simulink model "IPILCO_relativeRPY_ST"  (R2014b)
settings: Solver=ode45  StartTime=0.0  StopTime=T  RelTol=1e-3
values from neighbouring files (symbols this model uses):
  dt = 0.01    [settings_ST.m]    (also in settings_ST_puma.m)
  dt_pilco = 0.1    [settings_ST.m]    (also in settings_ST_puma.m)
  indices = 1:1:stateLength    [settings_ST.m]    (also in settings_ST_puma.m)
  initTrial = 0    [learnImp_ST.m]
  jj = J    [learnImp_ST.m]
  Kd_env = [1, 1, 0, 0, 0, 0]    [settings_ST.m]    (also in settings_ST_puma.m)
  Kp_env = [5e3, 5e3, 5e3, 0, 0, 0]    [settings_ST.m]    (also in settings_ST_puma.m = [4e3, 4e3, 0, 0, 0, 0])
  n = robot.n    [settings_ST.m]    (also in settings_ST_puma.m)
  perturbedRobotNF = perturbedRobot.nofriction('all')    [settings_ST.m]    (also in settings_ST_puma.m)
  robot = p560    [settings_ST.m]    (also in settings_ST_puma.m)
  seedMatrix = reshape(seedMatrix,J,[])    [settings_ST.m]    (also in settings_ST_puma.m)
  stateLength = 30    [settings_ST.m]    (also in settings_ST_puma.m)
  xc = [0.45, 0.45, 0.45, 10, 10, 10]'    [settings_ST.m]    (also in settings_ST_puma.m)
  xhole = [0.5, 0.1, 0]    [settings_ST.m]    (also in settings_ST_puma.m = [0.5, 0.2, 0])
undefined symbols (not defined in the file or in its folder): accel, addNoise, cardatol, computeDamping, Hd0, jacob0, jacob_dot, jacobn, plant, policy, q0, tr2rpy, transl, x0trial
libraries: roblocks x10, simulink x1, dspinverses x1
settings Model: Creator=LocalAdmin  LastModifiedBy=LocalAdmin

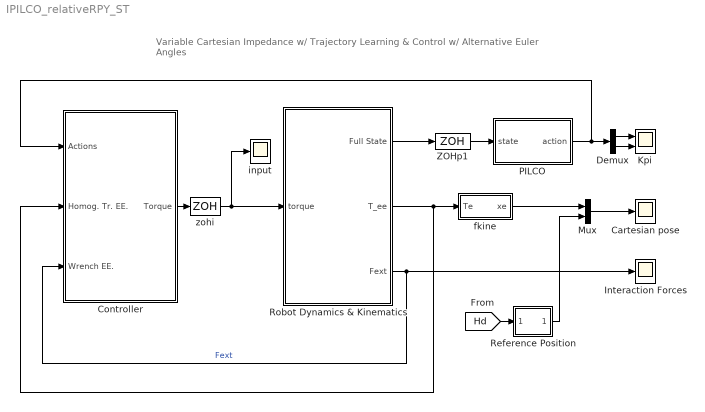
== system IPILCO_relativeRPY_ST ==
  note: Variable Cartesian Impedance w/ Trajectory Learning
      | & Control w/ Alternative Euler Angles
  Cartesian pose : Scope
      settings: TimeRange=0.05  YMin=-0.05  YMax=0.35
  Controller : Subsystem
  Demux : Demux  Outputs=2
  Interaction Forces : Scope
      settings: ShowLegends=on  TimeRange=5  YMin=-35  YMax=10  SaveName=ScopeData2
  Kpi : Scope  NumInputPorts=2
      settings: TimeRange=5  YMin=0~-0.002  YMax=250~0.006  SaveName=ScopeData3
  Mux : Mux  Inputs=2
  PILCO : Subsystem
  Reference Position : Subsystem
  Robot Dynamics & Kinematics : Subsystem
  ZOHp1 : ZeroOrderHold  SampleTime=dt
  fkine : Subsystem
  input : Scope
      settings: ShowLegends=on  TimeRange=0.13  YMin=-1500  YMax=1500  SaveName=ScopeData4
  zohi : ZeroOrderHold  SampleTime=dt
  wires:
  zohi/1 -> Robot Dynamics & Kinematics/1(torque), input/1
  Robot Dynamics & Kinematics/3(Fext) -> Controller/3(Wrench EE.), Interaction Forces/1  "Fext"
  Robot Dynamics & Kinematics/1(Full State) -> ZOHp1/1
  ZOHp1/1 -> PILCO/1(state)
  Controller/1(Torque) -> zohi/1
  Robot Dynamics & Kinematics/2(T_ee) -> Controller/2(Homog. Tr. EE.), fkine/1(Te)
  Reference Position/1(pd) -> Mux/2
  Mux/1 -> Cartesian pose/1
  PILCO/1(action) -> Demux/1, Controller/1(Actions)
  fkine/1(xe) -> Mux/1
  [Hd] -> Reference Position/1(Hd)
  Demux/1 -> Kpi/1
  Demux/2 -> Kpi/2

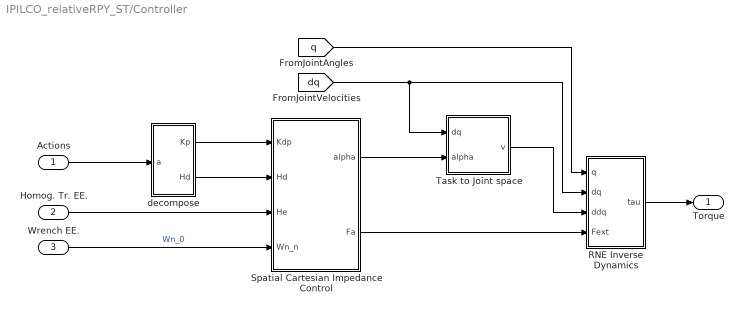
== system IPILCO_relativeRPY_ST/Controller ==
  Actions : Inport
  Homog. Tr. EE. : Inport  Port=2
  Wrench EE. : Inport  Port=3
  RNE Inverse Dynamics : Subsystem
  Spatial Cartesian Impedance Control : Subsystem
  Task to Joint space : Subsystem
  decompose : Subsystem
  Torque : Outport
  wires:
  Spatial Cartesian Impedance Control/1(alpha) -> Task to Joint space/2(alpha)
  Homog. Tr. EE./1 -> Spatial Cartesian Impedance Control/3(He)
  Wrench EE./1 -> Spatial Cartesian Impedance Control/4(Wn_n)  "Wn_0"
  Actions/1 -> decompose/1(a)
  decompose/1(Kp) -> Spatial Cartesian Impedance Control/1(Kdp)
  decompose/2(Hd) -> Spatial Cartesian Impedance Control/2(Hd)
  Task to Joint space/1(v) -> RNE Inverse Dynamics/3(ddq)
  RNE Inverse Dynamics/1(tau) -> Torque/1
  [dq] -> RNE Inverse Dynamics/2(dq), Task to Joint space/1(dq)
  Spatial Cartesian Impedance Control/2(Fa) -> RNE Inverse Dynamics/4(Fext)
  [q] -> RNE Inverse Dynamics/1(q)

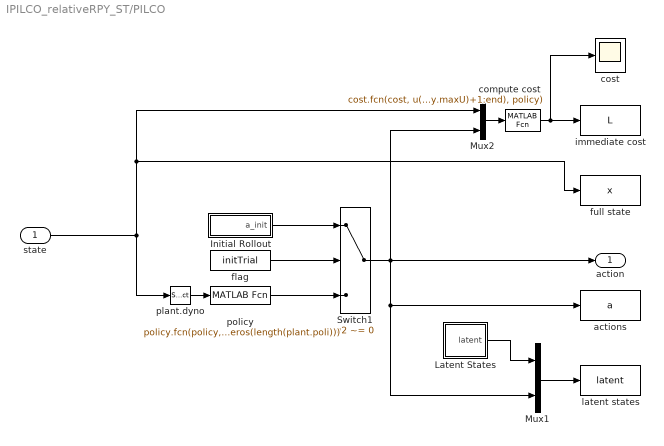
== system IPILCO_relativeRPY_ST/PILCO ==
  state : Inport
  Initial Rollout : Subsystem
  Latent States : Subsystem
  Mux1 : Mux  Inputs=2
  Mux2 : Mux  Inputs=2
  Switch1 : Switch  Criteria=u2 ~= 0
  actions : ToWorkspace  VariableName=a  SampleTime=dt_pilco
  compute cost : MATLABFcn  MATLABFcn=cost.fcn(cost, u(plant.dyno), zeros(length(plant.dyno)), u(end-length(policy.maxU)+1:end), policy)  OutputDimensions=1  Output1D=off
  cost : Scope
      settings: YMin=0  YMax=1.4
  flag : Constant  Value=initTrial  SampleTime=dt_pilco
  full state : ToWorkspace  VariableName=x  SampleTime=dt_pilco
  immediate cost : ToWorkspace  VariableName=L  SampleTime=dt_pilco
  latent states : ToWorkspace  VariableName=latent  SampleTime=dt_pilco
  plant.dyno : Selector  InputPortWidth=length(indices)  Indices=plant.dyno
  policy : MATLABFcn  MATLABFcn=policy.fcn(policy, u(plant.poli), zeros(length(plant.poli)))
  action : Outport
  wires:
  Mux1/1 -> latent states/1
  compute cost/1 -> cost/1, immediate cost/1
  plant.dyno/1 -> policy/1
  Mux2/1 -> compute cost/1
  state/1 -> full state/1, Mux2/1, plant.dyno/1
  Latent States/1(latent) -> Mux1/1
  flag/1 -> Switch1/2
  Initial Rollout/1(a_init) -> Switch1/1
  policy/1 -> Switch1/3
  Switch1/1 -> Mux2/2, Mux1/2, actions/1, action/1

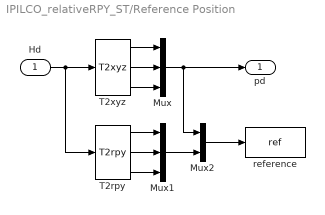
== system IPILCO_relativeRPY_ST/Reference Position ==
  Hd : Inport
  Mux : Mux  Inputs=3
  Mux1 : Mux  Inputs=3
  Mux2 : Mux  Inputs=2
  T2rpy : roblocks/Transform Conversion/T2rpy
  T2xyz : roblocks/Transform Conversion/T2xyz
  reference : ToWorkspace  VariableName=ref  SampleTime=dt_pilco
  pd : Outport
  wires:
  Hd/1 -> T2rpy/1, T2xyz/1
  T2xyz/1 -> Mux/1
  T2xyz/2 -> Mux/2
  T2xyz/3 -> Mux/3
  Mux/1 -> Mux2/1, pd/1
  T2rpy/1 -> Mux1/1
  T2rpy/2 -> Mux1/2
  T2rpy/3 -> Mux1/3
  Mux2/1 -> reference/1
  Mux1/1 -> Mux2/2

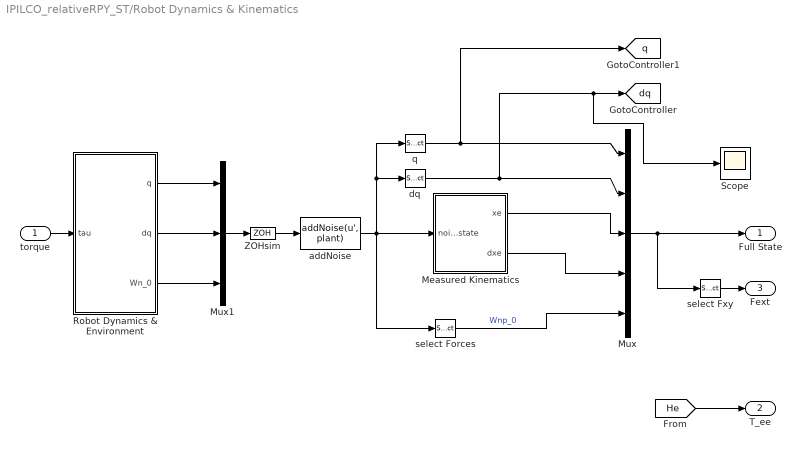
== system IPILCO_relativeRPY_ST/Robot Dynamics & Kinematics ==
  torque : Inport
  Measured Kinematics : Subsystem
  Mux : Mux  Inputs=5
  Mux1 : Mux  Inputs=3
  Robot Dynamics & Environment : Subsystem
  Scope : Scope
      settings: YMin=-80  YMax=60  SaveName=ScopeData7
  ZOHsim : ZeroOrderHold  SampleTime=dt
  addNoise : MATLABFcn  MATLABFcn=addNoise(u', plant)
  dq : Selector  InputPortWidth=2*robot.n+6  Indices=[robot.n+1:2*robot.n]
  q : Selector  InputPortWidth=2*robot.n+6  Indices=[1:robot.n]
  select Forces : Selector  InputPortWidth=2*robot.n+6  Indices=[2*robot.n+1:2*robot.n+6]
  select Fxy : Selector  InputPortWidth=stateLength  Indices=[stateLength-5:1:stateLength]
  Full State : Outport
  T_ee : Outport  Port=2
  Fext : Outport  Port=3
  tag scope: dq=global, q=global
  wires:
  torque/1 -> Robot Dynamics & Environment/1(tau)
  Measured Kinematics/1(xe) -> Mux/3
  Measured Kinematics/2(dxe) -> Mux/4
  select Fxy/1 -> Fext/1
  q/1 -> [q], Mux/1
  dq/1 -> Scope/1, [dq], Mux/2
  Robot Dynamics & Environment/1(q) -> Mux1/1
  Robot Dynamics & Environment/2(dq) -> Mux1/2
  Mux1/1 -> ZOHsim/1
  Robot Dynamics & Environment/3(Wn_0) -> Mux1/3
  Mux/1 -> Full State/1, select Fxy/1
  select Forces/1 -> Mux/5  "Wnp_0"
  [He] -> T_ee/1
  ZOHsim/1 -> addNoise/1
  addNoise/1 -> q/1, dq/1, select Forces/1, Measured Kinematics/1(noisy state)

== system IPILCO_relativeRPY_ST/fkine ==
  Te : Inport
  Mux1 : Mux  Inputs=6
  T2rpy : roblocks/Transform Conversion/T2rpy
  T2xyz : roblocks/Transform Conversion/T2xyz
  xe : Outport
  wires:
  Te/1 -> T2xyz/1, T2rpy/1
  T2xyz/2 -> Mux1/2
  T2rpy/1 -> Mux1/4
  T2xyz/1 -> Mux1/1
  T2rpy/2 -> Mux1/5
  Mux1/1 -> xe/1
  T2xyz/3 -> Mux1/3
  T2rpy/3 -> Mux1/6

== system IPILCO_relativeRPY_ST/Controller/RNE Inverse Dynamics ==
  q : Inport
  dq : Inport  Port=2
  ddq : Inport  Port=3
  Fext : Inport  Port=4
  Mux : Mux
  Recursive Newton-Euler : MATLABFcn  MATLABFcn=rne(robot.nofriction('all'), u(1:n)', u(n+1:2*n)', u(2*n+1:3*n)', robot.gravity', u(3*n+1:end)')  OutputDimensions=n
  tau : Outport
  wires:
  q/1 -> Mux/1
  dq/1 -> Mux/2
  ddq/1 -> Mux/3
  Fext/1 -> Mux/4
  Recursive Newton-Euler/1 -> tau/1
  Mux/1 -> Recursive Newton-Euler/1

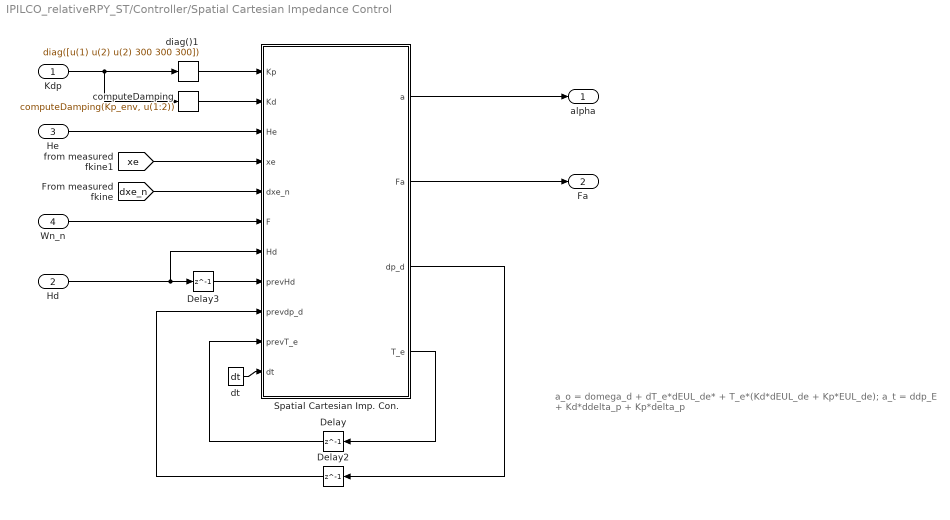
== system IPILCO_relativeRPY_ST/Controller/Spatial Cartesian Impedance Control ==
  note: a_o = domega_d + dT_e*dEUL_de* + T_e*(Kd*dEUL_de + Kp*EUL_de);
      |
      | a_t = ddp_E + Kd*ddelta_p + Kp*delta_p
  Kdp : Inport
  Hd : Inport  Port=2
  He : Inport  Port=3
  Wn_n : Inport  Port=4
  Delay : Delay  DelayLength=1  InitialCondition=cardatol(tr2rpy(Hd0),1,2,3)  SampleTime=dt
  Delay2 : Delay  DelayLength=1  InitialCondition=0  SampleTime=dt
  Delay3 : Delay  DelayLength=1  InitialCondition=Hd0  SampleTime=dt
  Spatial Cartesian Imp. Con. : MATLAB Function  TreatAsAtomicUnit=on
  computeDamping : MATLABFcn  MATLABFcn=computeDamping(Kp_env, u(1:2))  OutputDimensions=[6 6]  Output1D=off
  diag()1 : MATLABFcn  MATLABFcn=diag([u(1) u(2) u(2) 300 300 300])  OutputDimensions=[6 6]  Output1D=off
  dt : Constant  Value=dt  SampleTime=dt
  alpha : Outport
  Fa : Outport  Port=2
  wires:
  Spatial Cartesian Imp. Con./4(T_e) -> Delay/1
  Delay/1 -> Spatial Cartesian Imp. Con./10(prevT_e)
  dt/1 -> Spatial Cartesian Imp. Con./11(dt)
  Hd/1 -> Spatial Cartesian Imp. Con./7(Hd), Delay3/1
  He/1 -> Spatial Cartesian Imp. Con./3(He)
  diag()1/1 -> Spatial Cartesian Imp. Con./1(Kp)
  Spatial Cartesian Imp. Con./3(dp_d) -> Delay2/1
  Delay2/1 -> Spatial Cartesian Imp. Con./9(prevdp_d)
  Delay3/1 -> Spatial Cartesian Imp. Con./8(prevHd)
  [dxe_n] -> Spatial Cartesian Imp. Con./5(dxe_n)
  [xe] -> Spatial Cartesian Imp. Con./4(xe)
  Spatial Cartesian Imp. Con./1(a) -> alpha/1
  computeDamping/1 -> Spatial Cartesian Imp. Con./2(Kd)
  Kdp/1 -> computeDamping/1, diag()1/1
  Wn_n/1 -> Spatial Cartesian Imp. Con./6(F)
  Spatial Cartesian Imp. Con./2(Fa) -> Fa/1

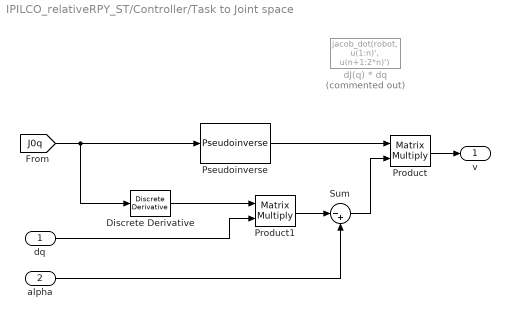
== system IPILCO_relativeRPY_ST/Controller/Task to Joint space ==
  dq : Inport
  alpha : Inport  Port=2
  Discrete Derivative : simulink/Discrete/Discrete Derivative  gainval=1.0  ICPrevScaledInput=0.0  InputProcessing=Inherited  OutMin=[]  OutMax=[]  OutDataType=fixdt(1, 16)  OutScaling=2^-10  DoSatur=off
  Product : Product  Multiplication=Matrix(*)
  Product1 : Product  Multiplication=Matrix(*)
  Pseudoinverse : dspinverses/Pseudoinverse  wanterr=off
  Sum : Sum  Inputs=|-+  SaturateOnIntegerOverflow=on  InputSameDT=on  OutDataTypeStr=Inherit: Same as first input
  dJ(q) * dq : MATLABFcn  Commented=on  MATLABFcn=jacob_dot(robot, u(1:n)', u(n+1:2*n)')  OutputDimensions=[6 1]  Output1D=off
  v : Outport
  wires:
  Discrete Derivative/1 -> Product1/1
  Sum/1 -> Product/2
  Product/1 -> v/1
  Pseudoinverse/1 -> Product/1
  alpha/1 -> Sum/2
  dq/1 -> Product1/2
  [J0q] -> Discrete Derivative/1, Pseudoinverse/1
  Product1/1 -> Sum/1

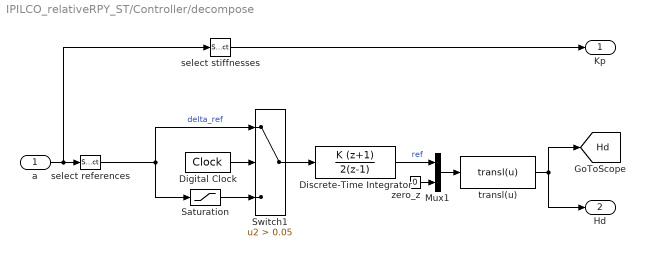
== system IPILCO_relativeRPY_ST/Controller/decompose ==
  a : Inport
  Digital Clock : DigitalClock  SampleTime=dt
  Discrete-Time Integrator : DiscreteIntegrator  IntegratorMethod=Accumulation: Trapezoidal  gainval=1  InitialCondition=x0trial(1:length(policy.refIdx))  InitialConditionSetting=State (most efficient)  SampleTime=-1  LimitOutput=on
  Mux1 : Mux  Inputs=2
  Saturation : Saturate  UpperLimit=0.001  LowerLimit=-0.001
  Switch1 : Switch  Criteria=u2 > Threshold  Threshold=0.05
  select references : Selector  InputPortWidth=length(policy.maxU)  Indices=policy.refIdx
  select stiffnesses : Selector  InputPortWidth=length(policy.maxU)  Indices=policy.impIdx
  transl(u) : MATLABFcn  MATLABFcn=transl(u)  OutputDimensions=[4 4]  Output1D=off
  zero_z : Constant  Value=0  SampleTime=dt
  Kp : Outport
  Hd : Outport  Port=2
  tag scope: Hd=global
  wires:
  select references/1 -> Switch1/1, Saturation/1  "delta_ref"
  select stiffnesses/1 -> Kp/1
  a/1 -> select references/1, select stiffnesses/1
  Discrete-Time Integrator/1 -> Mux1/1  "ref"
  zero_z/1 -> Mux1/2
  transl(u)/1 -> [Hd], Hd/1
  Mux1/1 -> transl(u)/1
  Switch1/1 -> Discrete-Time Integrator/1
  Digital Clock/1 -> Switch1/2
  Saturation/1 -> Switch1/3

== system IPILCO_relativeRPY_ST/PILCO/Initial Rollout ==
  Initial Pos. References : FromWorkspace  VariableName=ainit{jj}  SampleTime=dt  OutputAfterFinalValue=Holding final value
  Mux : Mux  Inputs=2
  Uniform Random Number : UniformRandomNumber  Minimum=policy.minU(policy.impIdx)  Maximum=policy.maxU(policy.impIdx).*2  Seed=seedMatrix(jj,:)  SampleTime=dt_pilco
  XY_des : Selector  InputPortWidth=6  Indices=[1 2]
  a_init : Outport
  wires:
  Initial Pos. References/1 -> XY_des/1
  Uniform Random Number/1 -> Mux/1
  Mux/1 -> a_init/1
  XY_des/1 -> Mux/2

== system IPILCO_relativeRPY_ST/PILCO/Latent States ==
  Mux : Mux  Inputs=5
  latent : Outport
  wires:
  [dq_latent] -> Mux/2
  [q_latent] -> Mux/1
  [wn_0_latent] -> Mux/5
  [dxe_latent] -> Mux/4
  [xe_latent] -> Mux/3
  Mux/1 -> latent/1

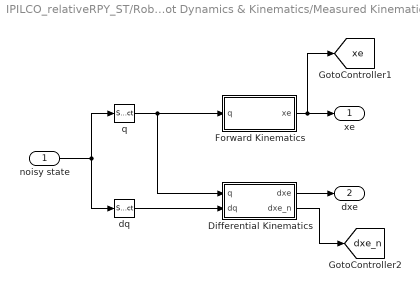
== system IPILCO_relativeRPY_ST/Robot Dynamics & Kinematics/Measured Kinematics ==
  noisy state : Inport
  Differential Kinematics : Subsystem
  Forward Kinematics : Subsystem
  dq : Selector  InputPortWidth=2*robot.n + 6  Indices=[robot.n+1:2*robot.n]
  q : Selector  InputPortWidth=2*robot.n+6  Indices=[1:robot.n]
  xe : Outport
  dxe : Outport  Port=2
  tag scope: dxe_n=global, xe=global
  wires:
  q/1 -> Differential Kinematics/1(q), Forward Kinematics/1(q)
  noisy state/1 -> q/1, dq/1
  dq/1 -> Differential Kinematics/2(dq)
  Differential Kinematics/1(dxe) -> dxe/1
  Forward Kinematics/1(xe) -> [xe], xe/1
  Differential Kinematics/2(dxe_n) -> [dxe_n]

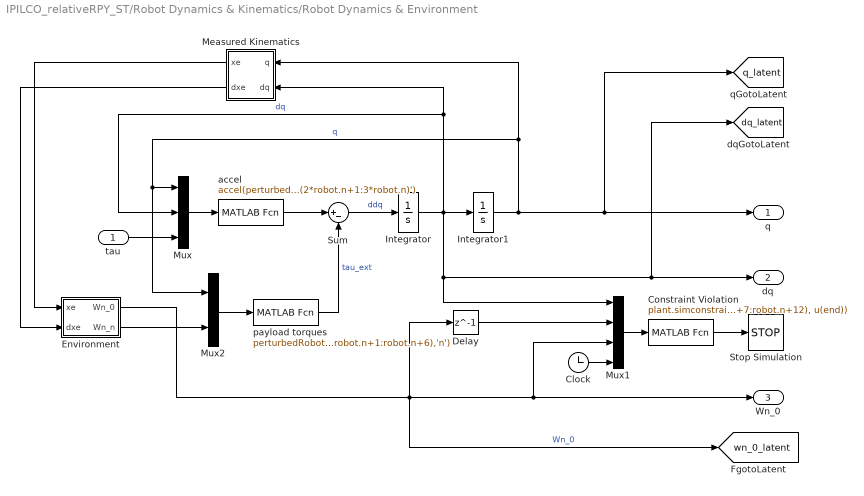
== system IPILCO_relativeRPY_ST/Robot Dynamics & Kinematics/Robot Dynamics & Environment ==
  tau : Inport
  Clock : Clock
  Constraint Violation : MATLABFcn  MATLABFcn=plant.simconstraint(u(1:robot.n), u(robot.n+1:robot.n+6), u(robot.n+7:robot.n+12), u(end))
  Delay : Delay  DelayLength=1  InitialCondition=0  SampleTime=dt
  Environment : Subsystem
  Integrator : Integrator
  Integrator1 : Integrator  InitialCondition=q0
  Measured Kinematics : Subsystem
  Mux : Mux  Inputs=3
  Mux1 : Mux
  Mux2 : Mux  Inputs=2
  Stop Simulation : Stop
  Sum : Sum  Inputs=|+-
  accel : MATLABFcn  MATLABFcn=accel(perturbedRobotNF,u(1:robot.n)',u(robot.n+1:2*robot.n)',u(2*robot.n+1:3*robot.n)')
  payload torques : MATLABFcn  MATLABFcn=perturbedRobotNF.pay(u(1:robot.n)',u(robot.n+1:robot.n+6),'n')
  q : Outport
  dq : Outport  Port=2
  Wn_0 : Outport  Port=3
  tag scope: dq_latent=global, q_latent=global, wn_0_latent=global
  wires:
  accel/1 -> Sum/1
  Mux/1 -> accel/1
  tau/1 -> Mux/3
  payload torques/1 -> Sum/2  "tau_ext"
  Sum/1 -> Integrator/1  "ddq"
  Mux1/1 -> Constraint Violation/1
  Constraint Violation/1 -> Stop Simulation/1
  Measured Kinematics/2(dxe) -> Environment/2(dxe)
  Integrator/1 -> Mux/2, Measured Kinematics/2(dq), Integrator1/1, Mux1/1, [dq_latent], dq/1  "dq"
  Integrator1/1 -> Measured Kinematics/1(q), Mux2/1, Mux/1, [q_latent], q/1  "q"
  Environment/1(Wn_0) -> Delay/1, [wn_0_latent], Mux1/3, Wn_0/1  "Wn_0"
  Mux2/1 -> payload torques/1
  Environment/2(Wn_n) -> Mux2/2
  Measured Kinematics/1(xe) -> Environment/1(xe)
  Delay/1 -> Mux1/2
  Clock/1 -> Mux1/4

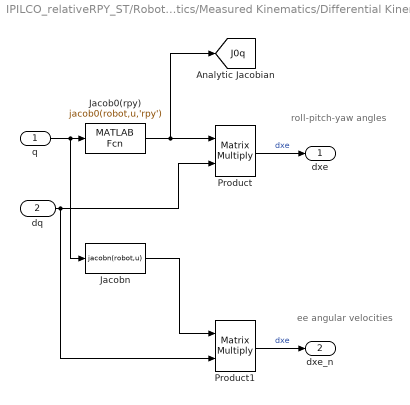
== system IPILCO_relativeRPY_ST/Robot Dynamics & Kinematics/Measured Kinematics/Differential Kinematics ==
  note: roll-pitch-yaw
      | angles
  note: ee angular
      | velocities
  q : Inport
  dq : Inport  Port=2
  Jacob0(rpy) : MATLABFcn  MATLABFcn=jacob0(robot,u,'rpy')  OutputDimensions=[6 n]  Output1D=off
  Jacobn : MATLABFcn  MATLABFcn=jacobn(robot,u)  OutputDimensions=[6 n]  Output1D=off
  Product : Product  Multiplication=Matrix(*)
  Product1 : Product  Multiplication=Matrix(*)
  dxe : Outport
  dxe_n : Outport  Port=2
  tag scope: J0q=global
  wires:
  q/1 -> Jacobn/1, Jacob0(rpy)/1
  Product/1 -> dxe/1  "dxe"
  Jacob0(rpy)/1 -> [J0q], Product/1
  Jacobn/1 -> Product1/1
  Product1/1 -> dxe_n/1  "dxe"
  dq/1 -> Product1/2, Product/2

== system IPILCO_relativeRPY_ST/Robot Dynamics & Kinematics/Measured Kinematics/Forward Kinematics ==
  q : Inport
  Mux : Mux  Inputs=6
  T2rpy : roblocks/Transform Conversion/T2rpy
  T2xyz : roblocks/Transform Conversion/T2xyz
  fkine : roblocks/Kinematics/fkine  robot=robot
  xe : Outport
  tag scope: He=global
  wires:
  T2xyz/3 -> Mux/3
  T2rpy/3 -> Mux/6
  T2rpy/1 -> Mux/4
  T2xyz/2 -> Mux/2
  q/1 -> fkine/1
  fkine/1 -> T2rpy/1, T2xyz/1, [He]
  T2xyz/1 -> Mux/1
  T2rpy/2 -> Mux/5
  Mux/1 -> xe/1

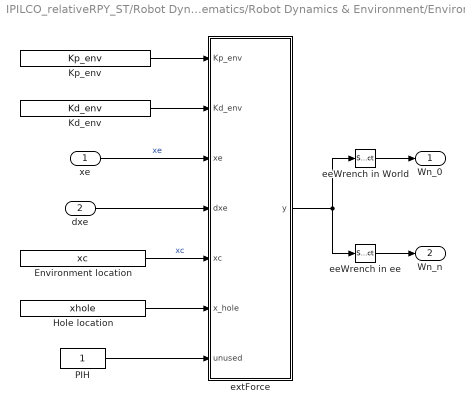
== system IPILCO_relativeRPY_ST/Robot Dynamics & Kinematics/Robot Dynamics & Environment/Environment ==
  xe : Inport
  dxe : Inport  Port=2
  Environment location : Constant  Value=xc  SampleTime=dt
  Hole location : Constant  Value=xhole  SampleTime=dt
  Kd_env : Constant  Value=Kd_env
  Kp_env : Constant  Value=Kp_env
  PIH : Constant  SampleTime=dt
  eeWrench in World : Selector  InputPortWidth=12  Indices=1:1:6
  eeWrench in ee : Selector  InputPortWidth=12  Indices=7:1:12
  extForce : MATLAB Function  TreatAsAtomicUnit=on
  Wn_0 : Outport
  Wn_n : Outport  Port=2
  wires:
  Environment location/1 -> extForce/5(xc)  "xc"
  xe/1 -> extForce/3(xe)  "xe"
  Kp_env/1 -> extForce/1(Kp_env)
  Kd_env/1 -> extForce/2(Kd_env)
  dxe/1 -> extForce/4(dxe)
  extForce/1(y) -> eeWrench in World/1, eeWrench in ee/1
  PIH/1 -> extForce/7(unused)
  eeWrench in World/1 -> Wn_0/1
  eeWrench in ee/1 -> Wn_n/1
  Hole location/1 -> extForce/6(x_hole)

== system IPILCO_relativeRPY_ST/Robot Dynamics & Kinematics/Robot Dynamics & Environment/Measured Kinematics ==
  q : Inport
  dq : Inport  Port=2
  Differential Kinematics : Subsystem
  Forward Kinematics : Subsystem
  xe : Outport
  dxe : Outport  Port=2
  tag scope: dxe_latent=global, xe_latent=global
  wires:
  q/1 -> Differential Kinematics/1(q), Forward Kinematics/1(q)
  dq/1 -> Differential Kinematics/2(dq)
  Differential Kinematics/1(dxe) -> [dxe_latent], dxe/1
  Forward Kinematics/1(xe) -> [xe_latent], xe/1

== system IPILCO_relativeRPY_ST/Robot Dynamics & Kinematics/Robot Dynamics & Environment/Measured Kinematics/Differential Kinematics ==
  q : Inport
  dq : Inport  Port=2
  Jacob0(rpy) : MATLABFcn  MATLABFcn=jacob0(robot,u,'rpy')  OutputDimensions=[6 n]  Output1D=off
  Product : Product  Multiplication=Matrix(*)
  dxe : Outport
  wires:
  q/1 -> Jacob0(rpy)/1
  Product/1 -> dxe/1  "dxe"
  dq/1 -> Product/2
  Jacob0(rpy)/1 -> Product/1

== system IPILCO_relativeRPY_ST/Robot Dynamics & Kinematics/Robot Dynamics & Environment/Measured Kinematics/Forward Kinematics ==
  q : Inport
  Mux : Mux  Inputs=6
  T2rpy : roblocks/Transform Conversion/T2rpy
  T2xyz : roblocks/Transform Conversion/T2xyz
  fkine : roblocks/Kinematics/fkine  robot=robot
  xe : Outport
  wires:
  T2xyz/3 -> Mux/3
  T2rpy/3 -> Mux/6
  T2rpy/1 -> Mux/4
  T2xyz/2 -> Mux/2
  q/1 -> fkine/1
  fkine/1 -> T2rpy/1, T2xyz/1
  T2xyz/1 -> Mux/1
  T2rpy/2 -> Mux/5
  Mux/1 -> xe/1

== matlab function IPILCO_relativeRPY_ST/Controller/Spatial Cartesian Impedance Control/Spatial Cartesian Imp. Con. ==
  data: a output size=[6 1]; Fa output size=[6 1]; dp_d output size=[3 1]; Kp input size=[6 6]; Kd input size=[6 6]; He input size=[4 4]; xe input size=[6 1]; dxe_n input size=[6 1]; F input size=[6 1]; Hd input size=[4 4]; prevHd input size=[4 4]; prevdp_d input size=[3 1]; prevT_e input size=[3 3]; T_e output size=[3 3]; dt input size=1
function [a, Fa, dp_d, T_e] = altEulCartImpControl(Kp, Kd, He, xe, dxe_n, F, Hd, prevHd, prevdp_d, prevT_e, dt)
% Computes modified euler angles EUL_de
%
% Outputs
%               - a             computed impedance actions in Cartesian space
%               - Ta            Transformation between analytical and geometric Jacobian
%               - T_e           transformation of Euler angle deriv. to angular vel. of ee-frame
%               - dT_e          time derivative of transf. matrix.
%
% Inputs:
%               - Kp                diagonal stiffness matrix
%               - Kd                diagonal damping matrix
%               - He                current homog. transf. of ee-frame
%               - Hd                desired homog. transf.
%               - xe                current end-effector pose
%               - dxe_n             current end-effector velocity (ee-frame
%               - prevHd            previous desired homog. transf.
%               - prevdp_d          previous desired translational velocity
%               - prevEUL_de        previous relative euler angles
%               - prevHe            previous homog. transf. of ee-frame
%               - dt                sampling time
%
% Code by Victor van Spaandonk
% May 2016
%

%% Prepare inputs
R_e = tr2rt(He);         % Rotation of ee-frame          (referred to base)
R_d = tr2rt(Hd);          % Rotation of desired frame     (referred to base)

Md = diag([1 1 1 1 1 1]);

%% Translational Actions
p_e = xe(1:3);                  % current ee pos.
p_d = transl(Hd);               % current desired pos.
delta_p = (p_d - p_e);          % positional error

dp_e = dxe_n(1:3);              % current ee transl vel.
prevp_d = transl(prevHd);       % previous desired postion
dp_d = (p_d - prevp_d)./dt;     % current desired velocity
ddelta_p = (dp_d - dp_e);       % velocity error

ddp_d = (dp_d - prevdp_d)./dt;  % current desired acceleration

a_t = ddp_d + inv(Md(1:3,1:3))*(Kd(1:3,1:3)*ddelta_p + Kp(1:3,1:3)*delta_p + F(1:3));

%% Rotational Actions
% EUL_e = my_tr2rpy(R_e,'xyz');           % Euler angles of ee-frame
% Te = cardatol(EUL_e,1,2,3);             % transformation between euler angles derivative and angular velocity of ee-frame
% Ta = [eye(3), zeros(3); zeros(3), Te];  % Transformation relating Geometric and Analytical Jacobian

Re_d = R_e'*R_d;                        % mutual orientation of ee-frame w.r.t. desired frame
EUL_de = my_tr2rpy(Re_d,'xyz')';        % extract EULER rpy-angles (xyz)

T = cardatol(EUL_de,1,2,3);             % Transformation matrix relating Euler angle derivatives to angular velocity      (xyz)
T_e = R_e*T;                            % Relative transformation referred to base-frame
dT_e = (T_e - prevT_e)./dt;             % time derivative of the transformation matrix  --> should not be numeric! TODO
Ta = [eye(3), zeros(3); zeros(3), T];  % Transformation relating Geometric and Analytical Jacobian of relative error frames

omega_e = dxe_n(4:6);                   % angular velocity of ee-frame
omega_d = [0;0;0];          % = tr2rt(Hd);% angular velocity of desired frame
deltaOmega_de = omega_d - omega_e;      % difference in ang. vel.
dEUL_de =  T_e\deltaOmega_de;           % derivative of relative Euler angles

domega_d = zeros(3,1);                  % desired angular velocity
a_o = domega_d + dT_e*dEUL_de + inv(Md(4:6,4:6))*T_e*(Kd(4:6,4:6)*dEUL_de + Kp(4:6,4:6)*EUL_de + (inv(T)')*F(4:6) );

Fa = inv(Ta)'*F;
a = [a_t; a_o];

== matlab function IPILCO_relativeRPY_ST/Robot Dynamics & Kinematics/Robot Dynamics & Environment/Environment/extForce ==
  data: Kp_env input; y output; Kd_env input; xe input; dxe input; xc input; x_hole input; unused input
function y = extForcefcn(Kp_env, Kd_env, xe, dxe, xc, x_hole, ~)
%Simulate external forces when performing PIH insertion.
% Environment is modelled as a spring+directional damping
%
% 1) Fext = Wrench on ee, expressed in perpendicular ee-frame
% 2) transform wrench from pee-frame to ee-frame
% 3) transform back to joints with geometric jacobian in ee-frame
%
%% Inits
persistent inHole INSERTED;
if isempty(inHole)
    inHole = 0;
end
if isempty(INSERTED)
    INSERTED = false;
end
Fext = zeros(6,1);  
contact = 0;

%% Constants
cf_v = 0;               % viscous friction coefficient
insertStiffness = 300;  % stiffness to overcome insertion.
r_hole = 0.005;          % tolerance per side of the peg
ywall_l = x_hole(2)+r_hole; ywall_r = x_hole(2)-r_hole;

%% Homogeneous Transformations
R0_n = my_rpy2r(xe(4:6)','xyz');    % roll-pitch-yaw angles of ee-frame w.r.t. base frame
p0_n = xe(1:3);
H0_n = rt2tr(R0_n,p0_n);                            % transform from world to ee-frame (fkine)

% H0_np = rt2tr(eye(3), xe(1:3));                     % homog. transf. from world-frame to ee-frame perpendicular to wall
% Hnp_0 = rt2tr(eye(3), -xe(1:3));
% Hnp_n = H0_n*Hnp_0;

%% determine state
% R0_np = eye(3);
% rpy = tr2diff(R0_np,R0_n);          % roll-pitch-yaw angles between base-frame and ee-frame
% rpy = xe(4:6);

if xe(1) > xc(1)
    contact = 1;
    if xe(2) > ywall_r && xe(2) < ywall_l %&& ((rpy(2)+rpy(3)) < 2*pi*(10/360))  % pitch+yaw should be less than 5 degrees
        inHole = 1;
    end
end

if xe(2) > xc(2)        % contact with surrounding box
    Fext(2) = Kp_env(2)*(xe(2)-xc(2));
elseif xe(2) < -xc(2)
    Fext(2) = Kp_env(2)*(-xe(2)-xc(2));
end

%% Insertion Forces
if contact && ~inHole            % wall contact

    Fext(1) = Kp_env(1)*(xe(1)-xc(1));              % stiffness force -X
    if dxe(1) > 0
        Fext(1) = Fext(1) + Kd_env(1)*dxe(1);       % damping force   -X
    end
    
%     Fn = cf_v * Fext(1);                    % normal force
%     Fext(2) = Fext(2) + Fn*sign(dxe(2));   % Coulomb friction +-Y
%     Fext(3) = Fext(3) + Fn*sign(dxe(3));   % Couloumb friction +-Z
    
    Fext(2) = Fext(2) + cf_v*dxe(2);   % viscous friction +-Y
    Fext(3) = Fext(3) + cf_v*dxe(3);   % viscous friction +-Z
    
elseif contact && inHole    % peg is in hole

    % end of hole        
    if xe(1) > x_hole(1) + 0.05;                    
        INSERTED = true;
        Fext(1) = Fext(1) + Kp_env(1)*(xe(1)-(x_hole(1) + 0.05)); % stiffness force -X
        if dxe(1) > 0
            Fext(1) = Fext(1) + Kd_env(1)*dxe(1);       % damping force   -X
        end
    end
    
    if xe(1) > x_hole(1)+0.016 && xe(1) < x_hole(1)+0.033 && ~INSERTED
        Fext(1) = Fext(1) + insertStiffness*(xe(1) - (x_hole(1)+0.016));   % insertion resistance -X
    end
    
    % Simulate walls:
    if xe(2) > ywall_l          %&& xe(1) < x_hole(1)+0.033                        
        Fext(2) = Fext(2) + Kp_env(2)*(xe(2)-ywall_l);            % perp. wall stiffness -Y
        if dxe(2) > 0
            Fext(2) = Fext(2) + Kd_env(2)*dxe(2);       % damping force   -Y
        end
        
        Fext(1) = Fext(1) + Fext(2)*cf_v*dxe(1);                  % friction force -X
        
    elseif xe(2) < ywall_r      % && xe(1) < x_hole(1)+0.033  
        Fext(2) = Fext(2) + Kp_env(2)*(xe(2)-ywall_r);  % perp. wall stiffness -Y
        if dxe(2) < 0
            Fext(2) = Fext(2) + Kd_env(2)*dxe(2);       % damping force   -Y
        end
        
        Fext(1) = Fext(1) + Fext(2)*cf_v*dxe(1);        % wall friction force -X
    end
end

W0_n = -Fext;                     % wrench in world frame
Wn_n = wtrans(H0_n, W0_n);       % wrench in ee-frame
y = [W0_n; Wn_n];
